simulink model "TestFilter"  (Simulink 6.6)
settings: Solver=ode45  StartTime=0.0  StopTime=10.0  RelTol=1e-3
undefined symbols (not defined in the file or in its folder): DiscIntNeverNeededParam, floatToBytes, gaind, polesd, u1, y1, zerosd
libraries: simulink x22, dsPICdrivers x15, aerolibguid x1, aerolibutil x1, dspmtrx3 x1
(part 1 of 2)
settings Model: Creator=ASL_Lab  LastModifiedBy=ASL_Lab

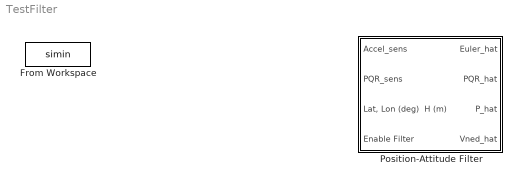
== system TestFilter ==
  From Workspace : FromWorkspace  VariableName=simin  SampleTime=0
  Position-Attitude Filter : Subsystem

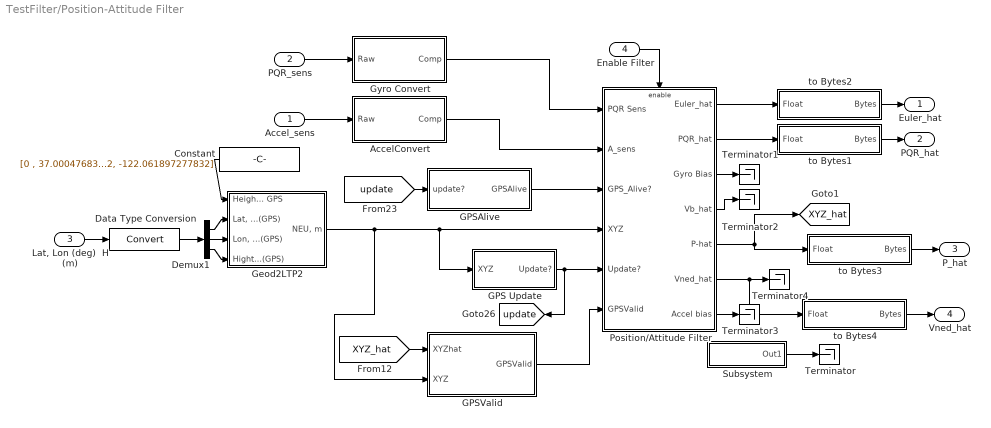
== system TestFilter/Position-Attitude Filter ==
  Accel_sens : Inport
  PQR_sens : Inport  Port=2
  "Lat, Lon (deg)  H (m)" : Inport  Port=3
  Enable Filter : Inport  Port=4
  AccelConvert : Subsystem  mask{bias=[2012 2018 2007], gains=[-41 41 -41]}
      mask prompts: bias "Initial Bias"; gains "Initial Gains"
      mask help: Convert Analog readings to units
  Constant : Constant  Orientation=left  Value=[0 , 37.0004768371582, -122.061897277832]
  Data Type Conversion : DataTypeConversion  OutDataTypeMode=double
  Demux1 : Demux  Outputs=3
  GPS Update : Subsystem  mask{T=0.01}
      mask prompts: T "Sample Time"
  GPSAlive : Subsystem  mask{deadLimit=4, T=0.01}
      mask prompts: deadLimit "Dead Limit (in Secs)"; T "Sample Time"
  GPSValid : Subsystem  mask{deadLimit=2000}
      mask prompts: deadLimit "Maximum Distance Error (in Mts)"
  Geod2LTP2 : Subsystem
      mask Description:
      | This block provides transformation of the Geodetic coordinates
      | to the LTP coorinate system. The block uses two consecutive transformations
      | (Geodetic -> ECEF ->LTP).
      | Geodetic coordinates of the LTP origin should also be predetermined.
      mask Help: Oops!
      mask Display: plot(0,0,100,100,[45,40,35,40,40],[85,95,85,95,40],[85,95,85,95,40],[35,40,45,40,40],[60,40,10,20,10,14],[70,40,10,13,10,20],[56,45],[70,70],[60,60],[50,60],[60,60],[30,40],[50,60],[20,20],[30,40],[20,20],[45,55],[35,25],[75,65],[35,25])
  Gyro Convert : Subsystem  mask{bias=[1863 2037 2040], gains=[-142 142 235]}
      mask prompts: bias "Initial Bias"; gains "Initial Gains"
      mask help: Convert Analog readings to units
  Position/Attitude Filter : Subsystem
  Subsystem : Subsystem
  Terminator{,1..4} (5 alike) : Terminator
  to Bytes1 : Subsystem
  to Bytes2 : Subsystem
  to Bytes3 : Subsystem
  to Bytes4 : Subsystem
  Euler_hat : Outport
  PQR_hat : Outport  Port=2
  P_hat : Outport  Port=3
  Vned_hat : Outport  Port=4
  tag scope: XYZ_hat=global, update=global
  wires:
  Enable Filter/1 -> Position/Attitude Filter/Enable
  Accel_sens/1 -> AccelConvert/1(Raw)
  PQR_sens/1 -> Gyro Convert/1(Raw)
  Geod2LTP2/1("NEU, m") -> GPS Update/1(XYZ), Position/Attitude Filter/4(XYZ), GPSValid/2(XYZ)
  "Lat, Lon (deg)  H (m)"/1 -> Data Type Conversion/1
  Demux1/3 -> Geod2LTP2/4(Hight,m(GPS))
  Demux1/2 -> Geod2LTP2/3("Lon, deg(GPS)")
  Demux1/1 -> Geod2LTP2/2("Lat, deg(GPS)")
  Constant/1 -> Geod2LTP2/1("Height, Lat, Lon Initials from GPS")
  GPSValid/1(GPSValid) -> Position/Attitude Filter/6(GPSValid)
  [XYZ_hat] -> GPSValid/1(XYZhat)
  GPSAlive/1(GPSAlive) -> Position/Attitude Filter/3(GPS_Alive?)
  [update] -> GPSAlive/1(update?)
  GPS Update/1(Update?) -> Position/Attitude Filter/5(Update?), [update]
  to Bytes2/1(Bytes) -> Euler_hat/1
  to Bytes1/1(Bytes) -> PQR_hat/1
  to Bytes3/1(Bytes) -> P_hat/1
  to Bytes4/1(Bytes) -> Vned_hat/1
  Subsystem/1(Out1) -> Terminator/1
  Position/Attitude Filter/5(P-hat) -> [XYZ_hat], to Bytes3/1(Float)
  Position/Attitude Filter/6(Vned_hat) -> Terminator4/1, to Bytes4/1(Float)
  Position/Attitude Filter/3(Gyro Bias) -> Terminator1/1
  Position/Attitude Filter/4(Vb_hat) -> Terminator2/1
  Position/Attitude Filter/7(Accel bias) -> Terminator3/1
  Position/Attitude Filter/1(Euler_hat) -> to Bytes2/1(Float)
  Position/Attitude Filter/2(PQR_hat) -> to Bytes1/1(Float)
  Gyro Convert/1(Comp) -> Position/Attitude Filter/1(PQR Sens)
  AccelConvert/1(Comp) -> Position/Attitude Filter/2(A_sens)
  Data Type Conversion/1 -> Demux1/1

== system TestFilter/Position-Attitude Filter/AccelConvert ==
  Raw : Inport
  Bias : Constant  Value=bias
  Divide : Product  Inputs=/*  OutScaling=2^-10
  Gains : Constant  Value=gains
  Sum : Sum  Inputs=|+-
  Comp : Outport
  wires:
  Raw/1 -> Sum/1
  Divide/1 -> Comp/1
  Sum/1 -> Divide/2
  Gains/1 -> Divide/1
  Bias/1 -> Sum/2

== system TestFilter/Position-Attitude Filter/GPS Update ==
  XYZ : Inport
  Demux : Demux  Outputs=3
  Detect Change : Subsystem
  Detect Change1 : Subsystem
  Detect Change2 : Subsystem
  Rate Transition : RateTransition  OutPortSampleTime=T
  Saturation1 : Saturate  UpperLimit=1  LowerLimit=0  SampleTime=T
  Sum : Sum  Inputs=3
  Update? : Outport
  wires:
  Rate Transition/1 -> Demux/1
  Saturation1/1 -> Update?/1
  XYZ/1 -> Rate Transition/1
  Sum/1 -> Saturation1/1
  Detect Change2/1(change?) -> Sum/3
  Detect Change1/1(change?) -> Sum/2
  Detect Change/1(change?) -> Sum/1
  Demux/3 -> Detect Change2/1(Data)
  Demux/2 -> Detect Change1/1(Data)
  Demux/1 -> Detect Change/1(Data)

== system TestFilter/Position-Attitude Filter/GPSAlive ==
  update? : Inport
  Compare To Constant : simulink/Logic and Bit Operations/Compare To Constant  SystemSampleTime=-1  relop=<=  const=deadLimit  LogicOutDataTypeMode=uint8  ZeroCross=off
  Constant : Constant
  Constant1 : Constant  Value=0
  Constant2 : Constant  Value=T
  Discrete-Time Integrator : DiscreteIntegrator  ExternalReset=rising  InitialConditionSource=external  SampleTime=T  ICPrevOutput=DiscIntNeverNeededParam  ICPrevScaledInput=DiscIntNeverNeededParam
  Integer Delay2 : simulink/Discrete/Integer Delay  vinit=0.0  samptime=-1  NumDelays=1
  Sum : Sum  Inputs=|++
  GPSAlive : Outport
  wires:
  Compare To Constant/1 -> GPSAlive/1
  Sum/1 -> Compare To Constant/1
  Constant2/1 -> Sum/2
  Integer Delay2/1 -> Sum/1
  update?/1 -> Discrete-Time Integrator/2
  Discrete-Time Integrator/1 -> Integer Delay2/1
  Constant1/1 -> Discrete-Time Integrator/3
  Constant/1 -> Discrete-Time Integrator/1

== system TestFilter/Position-Attitude Filter/GPSValid ==
  XYZhat : Inport
  XYZ : Inport  Port=2
  Calculate Range : aerolibguid/Calculate Range  SystemSampleTime=-1
  Compare To Constant : simulink/Logic and Bit Operations/Compare To Constant  SystemSampleTime=-1  relop=<=  const=deadLimit  LogicOutDataTypeMode=uint8  ZeroCross=off
  Integer Delay : simulink/Discrete/Integer Delay  vinit=0.0  samptime=0.01  NumDelays=1
  GPSValid : Outport
  wires:
  XYZ/1 -> Calculate Range/2
  Compare To Constant/1 -> GPSValid/1
  XYZhat/1 -> Integer Delay/1
  Calculate Range/1 -> Compare To Constant/1
  Integer Delay/1 -> Calculate Range/1

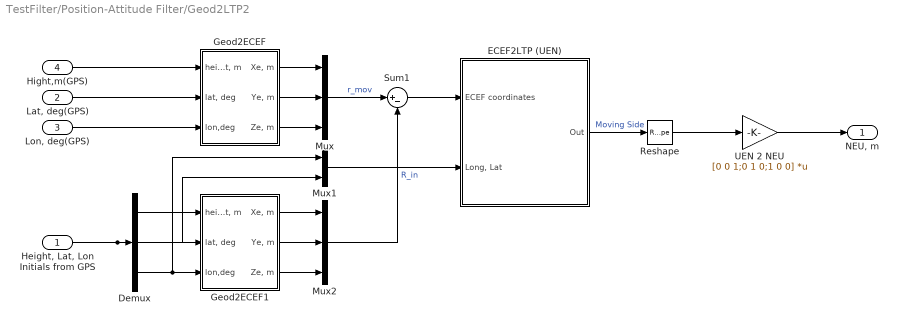
== system TestFilter/Position-Attitude Filter/Geod2LTP2 ==
  "Height, Lat, Lon Initials from GPS" : Inport
  "Lat, deg(GPS)" : Inport  Port=2
  "Lon, deg(GPS)" : Inport  Port=3
  Hight,m(GPS) : Inport  Port=4
  Demux : Demux  Outputs=3
  ECEF2LTP (UEN) : Subsystem
      mask Display: plot(0,0,100,100,[45,40,35,40,40],[85,95,85,95,40],[85,95,85,95,40],[35,40,45,40,40],[60,40,10,20,10,14],[70,40,10,13,10,20],[56,45],[70,70],[60,60],[50,60],[60,60],[30,40],[50,60],[20,20],[30,40],[20,20],[45,55],[35,25],[75,65],[35,25])
  Geod2ECEF : Subsystem  mask{Re=6378137, Rp=6356752.3142}
      mask prompts: Re "Enter equatorial radius, m"; Rp "Enter polar radius,m"
  Geod2ECEF1 : Subsystem  mask{Re=6378137, Rp=6356752.3142}
      mask prompts: Re "Enter equatorial radius, m"; Rp "Enter polar radius,m"
  Mux : Mux  Inputs=3
  Mux1 : Mux  Inputs=2
  Mux2 : Mux  Inputs=3
  Reshape : Reshape  OutputDimensionality=Column vector (2-D)
  Sum1 : Sum  Inputs=|+-  SaturateOnIntegerOverflow=on
  UEN 2 NEU : Gain  Gain=[0 0 1;0 1 0;1 0 0]  Multiplication=Matrix(K*u)  SaturateOnIntegerOverflow=on
  "NEU, m" : Outport
  wires:
  UEN 2 NEU/1 -> "NEU, m"/1
  Geod2ECEF/3("Ze, m ") -> Mux/3
  Geod2ECEF/1("Xe, m ") -> Mux/1
  Geod2ECEF/2("Ye, m ") -> Mux/2
  "Lat, deg(GPS)"/1 -> Geod2ECEF/2("lat, deg")
  "Lon, deg(GPS)"/1 -> Geod2ECEF/3(lon,deg)
  Mux1/1 -> ECEF2LTP (UEN)/2("Long, Lat")
  Geod2ECEF1/3("Ze, m ") -> Mux2/3
  Geod2ECEF1/1("Xe, m ") -> Mux2/1
  Geod2ECEF1/2("Ye, m ") -> Mux2/2
  Mux2/1 -> Sum1/2  "R_in"
  Demux/1 -> Geod2ECEF1/1("height, m")
  Demux/2 -> Mux1/2, Geod2ECEF1/2("lat, deg")
  Demux/3 -> Mux1/1, Geod2ECEF1/3(lon,deg)
  ECEF2LTP (UEN)/1(Out) -> Reshape/1  "Moving Side"
  Hight,m(GPS)/1 -> Geod2ECEF/1("height, m")
  "Height, Lat, Lon Initials from GPS"/1 -> Demux/1
  Mux/1 -> Sum1/1  "r_mov"
  Sum1/1 -> ECEF2LTP (UEN)/1(ECEF coordinates)
  Reshape/1 -> UEN 2 NEU/1

== system TestFilter/Position-Attitude Filter/Gyro Convert ==
  Raw : Inport
  Bias : Constant  Value=bias
  Divide : Product  Inputs=/*  OutScaling=2^-10
  Gains : Constant  Value=gains
  Sum : Sum  Inputs=|+-
  Comp : Outport
  wires:
  Bias/1 -> Sum/2
  Gains/1 -> Divide/1
  Sum/1 -> Divide/2
  Divide/1 -> Comp/1
  Raw/1 -> Sum/1

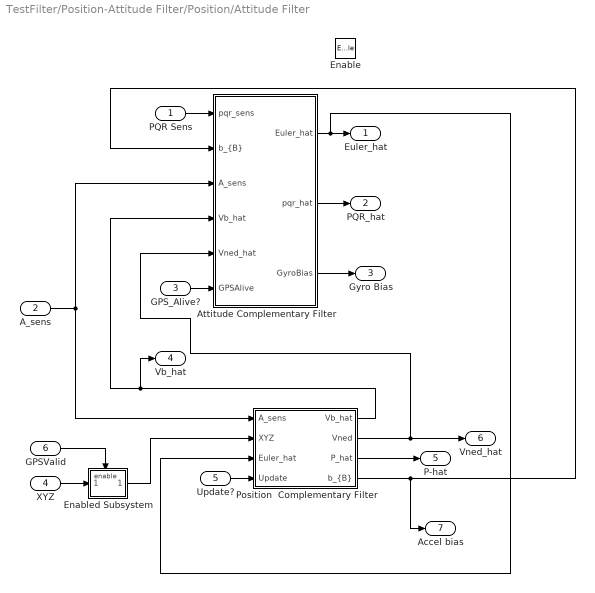
== system TestFilter/Position-Attitude Filter/Position/Attitude Filter ==
  PQR Sens : Inport
  A_sens : Inport  Port=2
  GPS_Alive? : Inport  Port=3
  XYZ : Inport  Port=4
  Update? : Inport  Port=5
  GPSValid : Inport  Port=6
  Enable : EnablePort  StatesWhenEnabling=reset
  Attitude Complementary Filter : Subsystem  mask{K1=0.7, K2=0.05, T=0.01, P0=[0 0 0], flpf=1}
      mask prompts: K1 "Euler Gain K1"; K2 "Bias Gain K2"; T "Filter Execution Time"; P0 "Initial Euler"; flpf "Feedback Low Pass Filter Freq (In S Domain)"
      mask help: Attitude Complementary filter based on the Magneto-Pendular Sensor by Vasconcelos, et.al.
      mask Help: Help
  Enabled Subsystem : Subsystem  TreatAsAtomicUnit=on
  Position  Complementary Filter : Subsystem  mask{K1=1.5, K2=0.5, K3=0.001, T=0.01, P0=[ 0 0 0], flpf=10}
      mask prompts: K1 "Position Gain K1"; K2 "Velocity Gain K2"; K3 "Bias Gain K3"; T "Filter Execution Time"; P0 "Initial Position"; flpf "Feedback Lowpass Filter Freq (in S domain)"
      mask help: Position Complementary filter based on the Magneto-Pendular Sensor by Vasconcelos, et.al.
      mask Help: Help
  Euler_hat : Outport
  PQR_hat : Outport  Port=2
  Gyro Bias : Outport  Port=3
  Vb_hat : Outport  Port=4
  P-hat : Outport  Port=5
  Vned_hat : Outport  Port=6
  Accel bias : Outport  Port=7
  wires:
  PQR Sens/1 -> Attitude Complementary Filter/1(pqr_sens)
  Attitude Complementary Filter/1(Euler_hat) -> Euler_hat/1, Position  Complementary Filter/3(Euler_hat)
  Attitude Complementary Filter/2(pqr_hat) -> PQR_hat/1
  A_sens/1 -> Attitude Complementary Filter/3(A_sens), Position  Complementary Filter/1(A_sens)
  Attitude Complementary Filter/3(GyroBias) -> Gyro Bias/1
  GPS_Alive?/1 -> Attitude Complementary Filter/6(GPSAlive)
  Position  Complementary Filter/1(Vb_hat) -> Attitude Complementary Filter/4(Vb_hat), Vb_hat/1
  Position  Complementary Filter/3(P_hat) -> P-hat/1
  Update?/1 -> Position  Complementary Filter/4(Update)
  Position  Complementary Filter/4("b_{B}") -> Accel bias/1, Attitude Complementary Filter/2("b_{B}")
  Position  Complementary Filter/2(Vned) -> Attitude Complementary Filter/5(Vned_hat), Vned_hat/1
  Enabled Subsystem/1(Out1) -> Position  Complementary Filter/2(XYZ)
  XYZ/1 -> Enabled Subsystem/1(In1)
  GPSValid/1 -> Enabled Subsystem/Enable

== system TestFilter/Position-Attitude Filter/Subsystem ==
  Mux : Mux  Inputs=3
  Sine Wave : Sin  SineType=Sample based  Amplitude=5*pi/180  Samples=100  SampleTime=.01
  Sine Wave1 : Sin  SineType=Sample based  Amplitude=10*pi/180  Samples=100  SampleTime=.01
  Sine Wave2 : Sin  SineType=Sample based  Amplitude=15*pi/180  Samples=100  SampleTime=.01
  Out1 : Outport
  wires:
  Sine Wave/1 -> Mux/1
  Sine Wave1/1 -> Mux/2
  Sine Wave2/1 -> Mux/3
  Mux/1 -> Out1/1

== system TestFilter/Position-Attitude Filter/to Bytes1 ==
  Float : Inport
  C Function Call : dsPICdrivers/OTHERS/C Function Call  Tag=dsPIC_dsPIC_CFunctionCall  fctName='floatToBytes'  INPUT_SIZE=1  INPUT1=real32  INPUT2=--  INPUT3=--  OUTPUT_SIZE=4  OUTPUT1=uint8  SampleTime=-1  InputType=[ 7 ]  OutputType=[ 2 ]  FctDeclaration=extern void floatToBytes(real32_T u1,uint8_T* y1);  FctCall=floatToBytes(%u1, *%y1);  OrderingInOutPopup=None
  C Function Call1 : dsPICdrivers/OTHERS/C Function Call  Tag=dsPIC_dsPIC_CFunctionCall  fctName='floatToBytes'  INPUT_SIZE=1  INPUT1=real32  INPUT2=--  INPUT3=--  OUTPUT_SIZE=4  OUTPUT1=uint8  SampleTime=-1  InputType=[ 7 ]  OutputType=[ 2 ]  FctDeclaration=extern void floatToBytes(real32_T u1,uint8_T* y1);  FctCall=floatToBytes(%u1, *%y1);  OrderingInOutPopup=None
  C Function Call2 : dsPICdrivers/OTHERS/C Function Call  Tag=dsPIC_dsPIC_CFunctionCall  fctName='floatToBytes'  INPUT_SIZE=1  INPUT1=real32  INPUT2=--  INPUT3=--  OUTPUT_SIZE=4  OUTPUT1=uint8  SampleTime=-1  InputType=[ 7 ]  OutputType=[ 2 ]  FctDeclaration=extern void floatToBytes(real32_T u1,uint8_T* y1);  FctCall=floatToBytes(%u1, *%y1);  OrderingInOutPopup=None
  Data Type Conversion : DataTypeConversion  OutDataTypeMode=single
  Demux : Demux  Outputs=3
  Mux : Mux  Inputs=3
  Bytes : Outport
  wires:
  Float/1 -> Data Type Conversion/1
  Demux/1 -> C Function Call/1
  Mux/1 -> Bytes/1
  C Function Call/1 -> Mux/1
  Demux/2 -> C Function Call1/1
  Demux/3 -> C Function Call2/1
  C Function Call1/1 -> Mux/2
  C Function Call2/1 -> Mux/3
  Data Type Conversion/1 -> Demux/1

== system TestFilter/Position-Attitude Filter/to Bytes2 ==
  Float : Inport
  C Function Call : dsPICdrivers/OTHERS/C Function Call  Tag=dsPIC_dsPIC_CFunctionCall  fctName='floatToBytes'  INPUT_SIZE=1  INPUT1=real32  INPUT2=--  INPUT3=--  OUTPUT_SIZE=4  OUTPUT1=uint8  SampleTime=-1  InputType=[ 7 ]  OutputType=[ 2 ]  FctDeclaration=extern void floatToBytes(real32_T u1,uint8_T* y1);  FctCall=floatToBytes(%u1, *%y1);  OrderingInOutPopup=None
  C Function Call1 : dsPICdrivers/OTHERS/C Function Call  Tag=dsPIC_dsPIC_CFunctionCall  fctName='floatToBytes'  INPUT_SIZE=1  INPUT1=real32  INPUT2=--  INPUT3=--  OUTPUT_SIZE=4  OUTPUT1=uint8  SampleTime=-1  InputType=[ 7 ]  OutputType=[ 2 ]  FctDeclaration=extern void floatToBytes(real32_T u1,uint8_T* y1);  FctCall=floatToBytes(%u1, *%y1);  OrderingInOutPopup=None
  C Function Call2 : dsPICdrivers/OTHERS/C Function Call  Tag=dsPIC_dsPIC_CFunctionCall  fctName='floatToBytes'  INPUT_SIZE=1  INPUT1=real32  INPUT2=--  INPUT3=--  OUTPUT_SIZE=4  OUTPUT1=uint8  SampleTime=-1  InputType=[ 7 ]  OutputType=[ 2 ]  FctDeclaration=extern void floatToBytes(real32_T u1,uint8_T* y1);  FctCall=floatToBytes(%u1, *%y1);  OrderingInOutPopup=None
  Data Type Conversion : DataTypeConversion  OutDataTypeMode=single
  Demux : Demux  Outputs=3
  Mux : Mux  Inputs=3
  Bytes : Outport
  wires:
  Data Type Conversion/1 -> Demux/1
  C Function Call2/1 -> Mux/3
  C Function Call1/1 -> Mux/2
  Demux/3 -> C Function Call2/1
  Demux/2 -> C Function Call1/1
  C Function Call/1 -> Mux/1
  Mux/1 -> Bytes/1
  Demux/1 -> C Function Call/1
  Float/1 -> Data Type Conversion/1

== system TestFilter/Position-Attitude Filter/to Bytes3 ==
  Float : Inport
  C Function Call : dsPICdrivers/OTHERS/C Function Call  Tag=dsPIC_dsPIC_CFunctionCall  fctName='floatToBytes'  INPUT_SIZE=1  INPUT1=real32  INPUT2=--  INPUT3=--  OUTPUT_SIZE=4  OUTPUT1=uint8  SampleTime=-1  InputType=[ 7 ]  OutputType=[ 2 ]  FctDeclaration=extern void floatToBytes(real32_T u1,uint8_T* y1);  FctCall=floatToBytes(%u1, *%y1);  OrderingInOutPopup=None
  C Function Call1 : dsPICdrivers/OTHERS/C Function Call  Tag=dsPIC_dsPIC_CFunctionCall  fctName='floatToBytes'  INPUT_SIZE=1  INPUT1=real32  INPUT2=--  INPUT3=--  OUTPUT_SIZE=4  OUTPUT1=uint8  SampleTime=-1  InputType=[ 7 ]  OutputType=[ 2 ]  FctDeclaration=extern void floatToBytes(real32_T u1,uint8_T* y1);  FctCall=floatToBytes(%u1, *%y1);  OrderingInOutPopup=None
  C Function Call2 : dsPICdrivers/OTHERS/C Function Call  Tag=dsPIC_dsPIC_CFunctionCall  fctName='floatToBytes'  INPUT_SIZE=1  INPUT1=real32  INPUT2=--  INPUT3=--  OUTPUT_SIZE=4  OUTPUT1=uint8  SampleTime=-1  InputType=[ 7 ]  OutputType=[ 2 ]  FctDeclaration=extern void floatToBytes(real32_T u1,uint8_T* y1);  FctCall=floatToBytes(%u1, *%y1);  OrderingInOutPopup=None
  Data Type Conversion : DataTypeConversion  OutDataTypeMode=single
  Demux : Demux  Outputs=3
  Mux : Mux  Inputs=3
  Bytes : Outport
  wires:
  Data Type Conversion/1 -> Demux/1
  C Function Call2/1 -> Mux/3
  C Function Call1/1 -> Mux/2
  Demux/3 -> C Function Call2/1
  Demux/2 -> C Function Call1/1
  C Function Call/1 -> Mux/1
  Mux/1 -> Bytes/1
  Demux/1 -> C Function Call/1
  Float/1 -> Data Type Conversion/1

== system TestFilter/Position-Attitude Filter/to Bytes4 ==
  Float : Inport
  C Function Call : dsPICdrivers/OTHERS/C Function Call  Tag=dsPIC_dsPIC_CFunctionCall  fctName='floatToBytes'  INPUT_SIZE=1  INPUT1=real32  INPUT2=--  INPUT3=--  OUTPUT_SIZE=4  OUTPUT1=uint8  SampleTime=-1  InputType=[ 7 ]  OutputType=[ 2 ]  FctDeclaration=extern void floatToBytes(real32_T u1,uint8_T* y1);  FctCall=floatToBytes(%u1, *%y1);  OrderingInOutPopup=None
  C Function Call1 : dsPICdrivers/OTHERS/C Function Call  Tag=dsPIC_dsPIC_CFunctionCall  fctName='floatToBytes'  INPUT_SIZE=1  INPUT1=real32  INPUT2=--  INPUT3=--  OUTPUT_SIZE=4  OUTPUT1=uint8  SampleTime=-1  InputType=[ 7 ]  OutputType=[ 2 ]  FctDeclaration=extern void floatToBytes(real32_T u1,uint8_T* y1);  FctCall=floatToBytes(%u1, *%y1);  OrderingInOutPopup=None
  C Function Call2 : dsPICdrivers/OTHERS/C Function Call  Tag=dsPIC_dsPIC_CFunctionCall  fctName='floatToBytes'  INPUT_SIZE=1  INPUT1=real32  INPUT2=--  INPUT3=--  OUTPUT_SIZE=4  OUTPUT1=uint8  SampleTime=-1  InputType=[ 7 ]  OutputType=[ 2 ]  FctDeclaration=extern void floatToBytes(real32_T u1,uint8_T* y1);  FctCall=floatToBytes(%u1, *%y1);  OrderingInOutPopup=None
  Data Type Conversion : DataTypeConversion  OutDataTypeMode=single
  Demux : Demux  Outputs=3
  Mux : Mux  Inputs=3
  Bytes : Outport
  wires:
  Float/1 -> Data Type Conversion/1
  Demux/1 -> C Function Call/1
  Mux/1 -> Bytes/1
  C Function Call/1 -> Mux/1
  Demux/2 -> C Function Call1/1
  Demux/3 -> C Function Call2/1
  C Function Call1/1 -> Mux/2
  C Function Call2/1 -> Mux/3
  Data Type Conversion/1 -> Demux/1

== system TestFilter/Position-Attitude Filter/GPS Update/Detect Change ==
  Data : Inport
  Abs1 : Abs  SampleTime=T
  Difference1 : simulink/Discrete/Difference  SystemSampleTime=-1  ICPrevInput=0.0  OutDataType=sfix(16)  OutScaling=2^-10  DoSatur=off
  Saturation1 : Saturate  UpperLimit=1  LowerLimit=0  SampleTime=T
  change? : Outport
  wires:
  Saturation1/1 -> change?/1
  Data/1 -> Difference1/1
  Abs1/1 -> Saturation1/1
  Difference1/1 -> Abs1/1

== system TestFilter/Position-Attitude Filter/GPS Update/Detect Change1 ==
  Data : Inport
  Abs1 : Abs  SampleTime=T
  Difference1 : simulink/Discrete/Difference  SystemSampleTime=-1  ICPrevInput=0.0  OutDataType=sfix(16)  OutScaling=2^-10  DoSatur=off
  Saturation1 : Saturate  UpperLimit=1  LowerLimit=0  SampleTime=T
  change? : Outport
  wires:
  Difference1/1 -> Abs1/1
  Abs1/1 -> Saturation1/1
  Data/1 -> Difference1/1
  Saturation1/1 -> change?/1

== system TestFilter/Position-Attitude Filter/GPS Update/Detect Change2 ==
  Data : Inport
  Abs1 : Abs  SampleTime=T
  Difference1 : simulink/Discrete/Difference  SystemSampleTime=-1  ICPrevInput=0.0  OutDataType=sfix(16)  OutScaling=2^-10  DoSatur=off
  Saturation1 : Saturate  UpperLimit=1  LowerLimit=0  SampleTime=T
  change? : Outport
  wires:
  Saturation1/1 -> change?/1
  Data/1 -> Difference1/1
  Abs1/1 -> Saturation1/1
  Difference1/1 -> Abs1/1

== system TestFilter/Position-Attitude Filter/Geod2LTP2/ECEF2LTP (UEN) ==
  ECEF coordinates : Inport
  "Long, Lat" : Inport  Port=2
  Deg2R : Gain  Gain=pi/180  SaturateOnIntegerOverflow=on
  Demux3 : Demux  Outputs=2
  From Body to Universal1 : Subsystem
  Product1 : Product  Multiplication=Matrix(*)  SaturateOnIntegerOverflow=on  InputSameDT=on
  Out : Outport
  wires:
  "Long, Lat"/1 -> Deg2R/1
  Product1/1 -> Out/1
  Demux3/2 -> From Body to Universal1/2(lat)
  Demux3/1 -> From Body to Universal1/1(long)
  Deg2R/1 -> Demux3/1
  ECEF coordinates/1 -> Product1/2
  From Body to Universal1/1(DCM) -> Product1/1

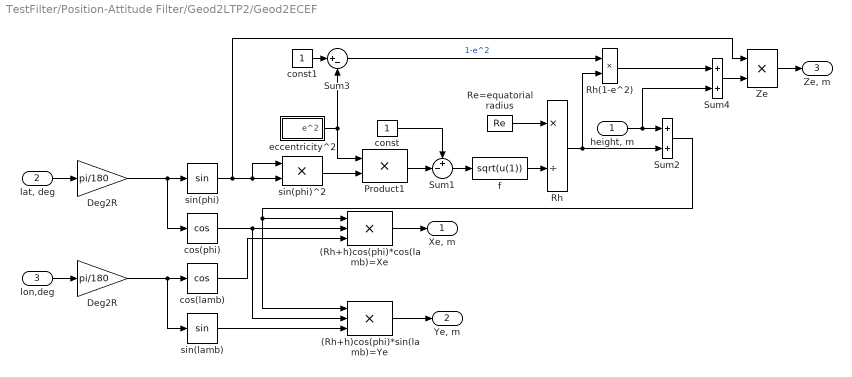
== system TestFilter/Position-Attitude Filter/Geod2LTP2/Geod2ECEF ==
  "height, m" : Inport
  "lat, deg" : Inport  Port=2
  lon,deg : Inport  Port=3
  (Rh+h)cos(phi)*cos(lamb)=Xe : Product  Inputs=3  SaturateOnIntegerOverflow=on  InputSameDT=on
  (Rh+h)cos(phi)*sin(lamb)=Ye : Product  Inputs=3  SaturateOnIntegerOverflow=on  InputSameDT=on
  Deg2R : Gain  Gain=pi/180  SaturateOnIntegerOverflow=on
  "Deg2R " : Gain  Gain=pi/180  SaturateOnIntegerOverflow=on
  Product1 : Product  SaturateOnIntegerOverflow=on  InputSameDT=on
  Re=equatorial radius : Constant  Value=Re
  Rh : Product  Inputs=*/  SaturateOnIntegerOverflow=on  InputSameDT=on
  Rh(1-e^2) : Product  SaturateOnIntegerOverflow=on  InputSameDT=on
  Sum1 : Sum  Inputs=+-|  SaturateOnIntegerOverflow=on  InputSameDT=on
  Sum2 : Sum  SaturateOnIntegerOverflow=on  InputSameDT=on
      settings: AttributesFormatString=Rh+h
  Sum3 : Sum  Inputs=|+-  SaturateOnIntegerOverflow=on  InputSameDT=on
  Sum4 : Sum  SaturateOnIntegerOverflow=on  InputSameDT=on
      settings: AttributesFormatString=(1-e^2)Rh+h
  Ze : Product  SaturateOnIntegerOverflow=on  InputSameDT=on
  const : Constant
  const1 : Constant
  cos(lamb) : Trigonometry  Operator=cos
  cos(phi) : Trigonometry  Operator=cos
  eccentricity^2 : Subsystem
  f : Fcn  Expr=sqrt(u(1))
  sin(lamb) : Trigonometry
  sin(phi) : Trigonometry
  sin(phi)^2 : Product  SaturateOnIntegerOverflow=on  InputSameDT=on
  "Xe, m " : Outport
  "Ye, m " : Outport  Port=2
  "Ze, m " : Outport  Port=3
  wires:
  "lat, deg"/1 -> Deg2R/1
  sin(phi)/1 -> sin(phi)^2/1, sin(phi)^2/2, Ze/1
  f/1 -> Rh/2
  Re=equatorial radius/1 -> Rh/1
  Rh/1 -> Sum2/2, Rh(1-e^2)/2
  Product1/1 -> Sum1/2
  Sum1/1 -> f/1
  const/1 -> Sum1/1
  "height, m"/1 -> Sum4/2, Sum2/1
  eccentricity^2/1(e^2) -> Product1/1, Sum3/2
  sin(phi)^2/1 -> Product1/2
  const1/1 -> Sum3/1
  Sum3/1 -> Rh(1-e^2)/1  "1-e^2"
  Rh(1-e^2)/1 -> Sum4/1
  Sum4/1 -> Ze/2
  lon,deg/1 -> "Deg2R "/1
  cos(phi)/1 -> (Rh+h)cos(phi)*cos(lamb)=Xe/2, (Rh+h)cos(phi)*sin(lamb)=Ye/2
  cos(lamb)/1 -> (Rh+h)cos(phi)*cos(lamb)=Xe/3
  sin(lamb)/1 -> (Rh+h)cos(phi)*sin(lamb)=Ye/3
  Ze/1 -> "Ze, m "/1
  Deg2R/1 -> cos(phi)/1, sin(phi)/1
  "Deg2R "/1 -> cos(lamb)/1, sin(lamb)/1
  Sum2/1 -> (Rh+h)cos(phi)*sin(lamb)=Ye/1, (Rh+h)cos(phi)*cos(lamb)=Xe/1
  (Rh+h)cos(phi)*cos(lamb)=Xe/1 -> "Xe, m "/1
  (Rh+h)cos(phi)*sin(lamb)=Ye/1 -> "Ye, m "/1

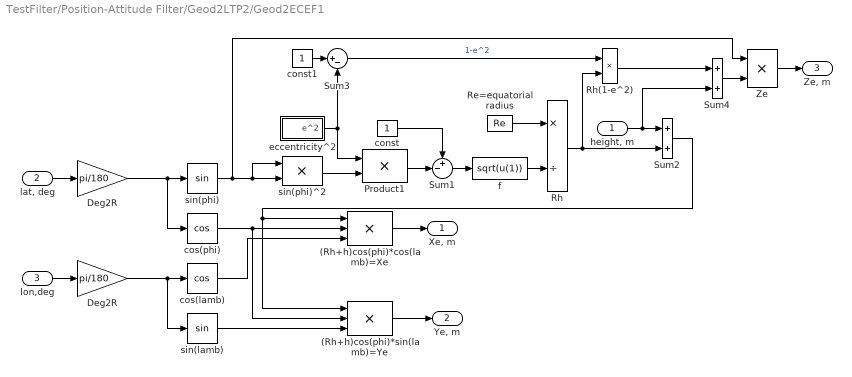
== system TestFilter/Position-Attitude Filter/Geod2LTP2/Geod2ECEF1 ==
  "height, m" : Inport
  "lat, deg" : Inport  Port=2
  lon,deg : Inport  Port=3
  (Rh+h)cos(phi)*cos(lamb)=Xe : Product  Inputs=3  SaturateOnIntegerOverflow=on  InputSameDT=on
  (Rh+h)cos(phi)*sin(lamb)=Ye : Product  Inputs=3  SaturateOnIntegerOverflow=on  InputSameDT=on
  Deg2R : Gain  Gain=pi/180  SaturateOnIntegerOverflow=on
  "Deg2R " : Gain  Gain=pi/180  SaturateOnIntegerOverflow=on
  Product1 : Product  SaturateOnIntegerOverflow=on  InputSameDT=on
  Re=equatorial radius : Constant  Value=Re
  Rh : Product  Inputs=*/  SaturateOnIntegerOverflow=on  InputSameDT=on
  Rh(1-e^2) : Product  SaturateOnIntegerOverflow=on  InputSameDT=on
  Sum1 : Sum  Inputs=+-|  SaturateOnIntegerOverflow=on  InputSameDT=on
  Sum2 : Sum  SaturateOnIntegerOverflow=on  InputSameDT=on
      settings: AttributesFormatString=Rh+h
  Sum3 : Sum  Inputs=|+-  SaturateOnIntegerOverflow=on  InputSameDT=on
  Sum4 : Sum  SaturateOnIntegerOverflow=on  InputSameDT=on
      settings: AttributesFormatString=(1-e^2)Rh+h
  Ze : Product  SaturateOnIntegerOverflow=on  InputSameDT=on
  const : Constant
  const1 : Constant
  cos(lamb) : Trigonometry  Operator=cos
  cos(phi) : Trigonometry  Operator=cos
  eccentricity^2 : Subsystem
  f : Fcn  Expr=sqrt(u(1))
  sin(lamb) : Trigonometry
  sin(phi) : Trigonometry
  sin(phi)^2 : Product  SaturateOnIntegerOverflow=on  InputSameDT=on
  "Xe, m " : Outport
  "Ye, m " : Outport  Port=2
  "Ze, m " : Outport  Port=3
  wires:
  (Rh+h)cos(phi)*sin(lamb)=Ye/1 -> "Ye, m "/1
  (Rh+h)cos(phi)*cos(lamb)=Xe/1 -> "Xe, m "/1
  Sum2/1 -> (Rh+h)cos(phi)*cos(lamb)=Xe/1, (Rh+h)cos(phi)*sin(lamb)=Ye/1
  "Deg2R "/1 -> sin(lamb)/1, cos(lamb)/1
  Deg2R/1 -> sin(phi)/1, cos(phi)/1
  Ze/1 -> "Ze, m "/1
  sin(lamb)/1 -> (Rh+h)cos(phi)*sin(lamb)=Ye/3
  cos(lamb)/1 -> (Rh+h)cos(phi)*cos(lamb)=Xe/3
  cos(phi)/1 -> (Rh+h)cos(phi)*sin(lamb)=Ye/2, (Rh+h)cos(phi)*cos(lamb)=Xe/2
  lon,deg/1 -> "Deg2R "/1
  Sum4/1 -> Ze/2
  Rh(1-e^2)/1 -> Sum4/1
  Sum3/1 -> Rh(1-e^2)/1  "1-e^2"
  const1/1 -> Sum3/1
  sin(phi)^2/1 -> Product1/2
  eccentricity^2/1(e^2) -> Sum3/2, Product1/1
  "height, m"/1 -> Sum2/1, Sum4/2
  const/1 -> Sum1/1
  Sum1/1 -> f/1
  Product1/1 -> Sum1/2
  Rh/1 -> Rh(1-e^2)/2, Sum2/2
  Re=equatorial radius/1 -> Rh/1
  f/1 -> Rh/2
  sin(phi)/1 -> Ze/1, sin(phi)^2/2, sin(phi)^2/1
  "lat, deg"/1 -> Deg2R/1

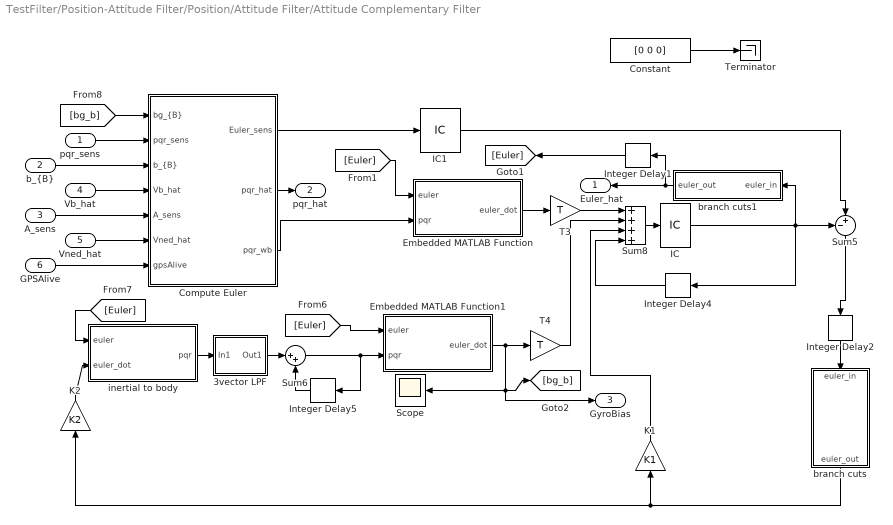
== system TestFilter/Position-Attitude Filter/Position/Attitude Filter/Attitude Complementary Filter ==
  pqr_sens : Inport
  "b_{B}" : Inport  Port=2
  A_sens : Inport  Port=3
  Vb_hat : Inport  Port=4
  Vned_hat : Inport  Port=5
  GPSAlive : Inport  Port=6
  3vector LPF : Subsystem  mask{flpf=flpf, T=T}
      mask prompts: flpf "Low Pass Frequency (in S domain)"; T "Sample time"
      mask Display: droots([],-flpf,flpf)
  Compute Euler : Subsystem
  Constant : Constant  Value=[0 0 0]
  Embedded MATLAB Function : Stateflow chart
  Embedded MATLAB Function1 : Stateflow chart
  IC : InitialCondition  Value=P0  SampleTime=T
  IC1 : InitialCondition  Value=P0  SampleTime=T
  Integer Delay1 : simulink/Discrete/Integer Delay  Orientation=left  vinit=0.0  samptime=-1  NumDelays=1
  Integer Delay2 : simulink/Discrete/Integer Delay  Orientation=down  vinit=0.0  samptime=-1  NumDelays=1
  Integer Delay4 : simulink/Discrete/Integer Delay  Orientation=left  vinit=0.0  samptime=-1  NumDelays=1
  Integer Delay5 : simulink/Discrete/Integer Delay  Orientation=left  vinit=0.0  samptime=-1  NumDelays=1
  K1 : Gain  Orientation=up  Gain=K1
  K2 : Gain  Orientation=up  Gain=K2
  Scope : Scope
      settings: TimeRange=60  YMin=-0.07116438310879042  YMax=0.01417979172834782  SaveName=ScopeData13
  Sum5 : Sum  Orientation=down  Inputs=-+|
  Sum6 : Sum  Inputs=|++
  Sum8 : Sum  Inputs=4
  T3 : Gain  Gain=T  SampleTime=T
  T4 : Gain  Gain=T  SampleTime=T
  Terminator : Terminator
  branch cuts : Stateflow chart  Orientation=down
  branch cuts1 : Stateflow chart  Orientation=left
  inertial to body : Stateflow chart
  Euler_hat : Outport  Orientation=left
  pqr_hat : Outport  Port=2
  GyroBias : Outport  Port=3
  wires:
  Embedded MATLAB Function/1(euler_dot) -> T3/1
  T3/1 -> Sum8/1
  Sum8/1 -> IC/1
  Integer Delay4/1 -> Sum8/4
  K1/1 -> Sum8/3
  inertial to body/1(pqr) -> 3vector LPF/1(In1)
  Sum6/1 -> Embedded MATLAB Function1/2(pqr), Integer Delay5/1
  [Euler] -> Embedded MATLAB Function1/1(euler)
  [Euler] -> inertial to body/1(euler)
  Embedded MATLAB Function1/1(euler_dot) -> [bg_b], Scope/1, GyroBias/1, T4/1
  T4/1 -> Sum8/2
  Integer Delay5/1 -> Sum6/2
  K2/1 -> inertial to body/2(euler_dot)
  [bg_b] -> Compute Euler/1("bg_{B}")
  pqr_sens/1 -> Compute Euler/2(pqr_sens)
  "b_{B}"/1 -> Compute Euler/3("b_{B}")
  Vb_hat/1 -> Compute Euler/4(Vb_hat)
  A_sens/1 -> Compute Euler/5(A_sens)
  Vned_hat/1 -> Compute Euler/6(Vned_hat)
  Sum5/1 -> Integer Delay2/1
  IC/1 -> Integer Delay4/1, Sum5/1, branch cuts1/1(euler_in)
  Integer Delay1/1 -> [Euler]
  [Euler] -> Embedded MATLAB Function/1(euler)
  Integer Delay2/1 -> branch cuts/1(euler_in)
  Compute Euler/3(pqr_wb) -> Embedded MATLAB Function/2(pqr)
  Compute Euler/2(pqr_hat) -> pqr_hat/1
  branch cuts/1(euler_out) -> K2/1, K1/1
  branch cuts1/1(euler_out) -> Euler_hat/1, Integer Delay1/1
  GPSAlive/1 -> Compute Euler/7(gpsAlive)
  3vector LPF/1(Out1) -> Sum6/1
  Compute Euler/1(Euler_sens) -> IC1/1
  IC1/1 -> Sum5/2
  Constant/1 -> Terminator/1

== system TestFilter/Position-Attitude Filter/Position/Attitude Filter/Enabled Subsystem ==
  In1 : Inport
  Enable : EnablePort
  Out1 : Outport
  wires:
  In1/1 -> Out1/1

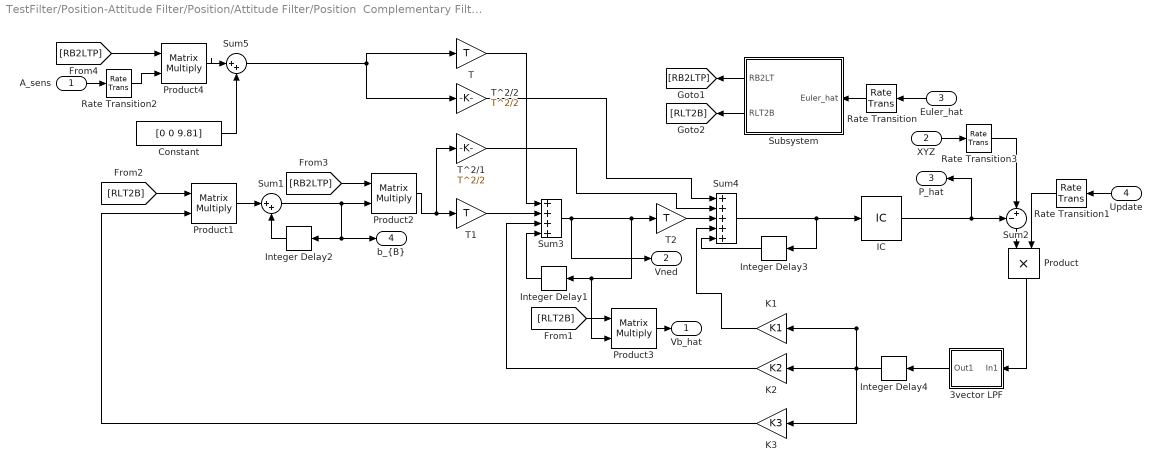
== system TestFilter/Position-Attitude Filter/Position/Attitude Filter/Position  Complementary Filter ==
  A_sens : Inport
  XYZ : Inport  Port=2
  Euler_hat : Inport  Orientation=left  Port=3
  Update : Inport  Orientation=left  Port=4
  3vector LPF : Subsystem  Orientation=left  mask{flpf=flpf, T=T}
      mask prompts: flpf "Low Pass Frequency (in S domain)"; T "Sample time"
      mask Display: droots([],-flpf,flpf)
  Constant : Constant  Value=[0 0 9.81]  SampleTime=0.01
  IC : InitialCondition  Value=P0  SampleTime=T
  Integer Delay{1..4} (4 alike) : simulink/Discrete/Integer Delay  Orientation=left  vinit=0.0  samptime=-1  NumDelays=1
  K1 : Gain  Orientation=left  Gain=K1
  K2 : Gain  Orientation=left  Gain=K2
  K3 : Gain  Orientation=left  Gain=K3
  Product : Product  Orientation=down  RndMeth=Zero
  Product{1..4} (4 alike) : Product  Multiplication=Matrix(*)  RndMeth=Zero
  Rate Transition : RateTransition  Orientation=left  OutPortSampleTime=T
  Rate Transition1 : RateTransition  Orientation=left  OutPortSampleTime=T
  Rate Transition2 : RateTransition  OutPortSampleTime=T
  Rate Transition3 : RateTransition  OutPortSampleTime=T
  Subsystem : Subsystem  Orientation=left
  Sum1 : Sum  Inputs=|++
  Sum2 : Sum  Orientation=down  Inputs=-+|
  Sum3 : Sum  Inputs=4
  Sum4 : Sum  Inputs=5
  Sum5 : Sum  Inputs=|++
  T : Gain  Gain=T
  T1 : Gain  Gain=T
  T2 : Gain  Gain=T
  T^2/1 : Gain  Gain=T^2/2
  T^2/2 : Gain  Gain=T^2/2
  Vb_hat : Outport
  Vned : Outport  Port=2
  P_hat : Outport  Orientation=left  Port=3
  "b_{B}" : Outport  Port=4
  wires:
  Subsystem/2(RLT2B) -> [RLT2B]
  Subsystem/1(RB2LT) -> [RB2LTP]
  Euler_hat/1 -> Rate Transition/1
  K3/1 -> Product1/2
  Product1/1 -> Sum1/1
  Sum1/1 -> Product2/2, Integer Delay2/1, "b_{B}"/1
  Product2/1 -> T^2/1/1, T1/1
  T1/1 -> Sum3/2
  T/1 -> Sum3/1
  Sum3/1 -> T2/1, Integer Delay1/1, Product3/2, Vned/1
  K2/1 -> Sum3/3
  T2/1 -> Sum4/3
  T^2/1/1 -> Sum4/2
  T^2/2/1 -> Sum4/1
  Sum4/1 -> Integer Delay3/1, IC/1
  K1/1 -> Sum4/4
  XYZ/1 -> Rate Transition3/1
  Product3/1 -> Vb_hat/1
  Sum2/1 -> Product/1
  Product/1 -> 3vector LPF/1(In1)
  Update/1 -> Rate Transition1/1
  Integer Delay3/1 -> Sum4/5
  Integer Delay2/1 -> Sum1/2
  Integer Delay1/1 -> Sum3/4
  A_sens/1 -> Rate Transition2/1
  Product4/1 -> Sum5/1
  Constant/1 -> Sum5/2
  Sum5/1 -> T/1, T^2/2/1
  Rate Transition/1 -> Subsystem/1(Euler_hat)
  Rate Transition1/1 -> Product/2
  Rate Transition3/1 -> Sum2/2
  [RLT2B] -> Product1/1
  [RB2LTP] -> Product4/1
  Rate Transition2/1 -> Product4/2
  [RB2LTP] -> Product2/1
  [RLT2B] -> Product3/1
  IC/1 -> Sum2/1, P_hat/1
  Integer Delay4/1 -> K1/1, K2/1, K3/1
  3vector LPF/1(Out1) -> Integer Delay4/1

== system TestFilter/Position-Attitude Filter/Geod2LTP2/ECEF2LTP (UEN)/From Body to Universal1 ==
  long : Inport
  lat : Inport  Port=2
  Mux : Mux  Inputs=2
  Reshape 9x1->3x1 : S-Function  FunctionName=sreshape  Parameters=OutputDimensionality, OutputDimensions  mask(Reshape){OutputDimensionality=Customize, OutputDimensions=[3,3]}
      mask prompts: OutputDimensionality "Output dimensionality:"; OutputDimensions "Output dimensions:"
      mask help:
      | Change the dimensions of a vector or matrix input signal. Output
      |  - a one-dimensional array (vector),
      |  - a column vector (Mx1 matrix),
      |  - a row vector (1xN matrix), or
      |  - a matrix or vector with specified dimensions, e.g., [M, N] or [W].
      mask init:
      | s = reshapemask(gcb,'init');
      mask StyleString: popup(1-D array|Column vector|Row vector|Customize),edit
      mask CallbackString: reshapemask(gcb,'cbDimensionality')|
      mask Display: disp('Reshape')
  Rotation Matrix from Long//Lat : Subsystem
      mask Type: Vector Transformation
      mask Description: Vector Transformation
      mask Display: disp('axis')
  DCM : Outport
  wires:
  lat/1 -> Mux/2
  long/1 -> Mux/1
  Mux/1 -> Rotation Matrix from Long//Lat/1(long lat)
  Rotation Matrix from Long//Lat/1(DCM) -> Reshape 9x1->3x1/1
  Reshape 9x1->3x1/1 -> DCM/1

== system TestFilter/Position-Attitude Filter/Geod2LTP2/Geod2ECEF/eccentricity^2 ==
  " " : Product  SaturateOnIntegerOverflow=on  InputSameDT=on
  Re=equatorial radius1 : Constant  Value=Re
  Rp=polar radius : Constant  Value=Rp
  Sum5 : Sum  Inputs=|+-  SaturateOnIntegerOverflow=on  InputSameDT=on
  const2 : Constant
  e^1 : Product  Inputs=*/  SaturateOnIntegerOverflow=on  InputSameDT=on
  e^2 : Outport
  wires:
  Re=equatorial radius1/1 -> e^1/2
  Rp=polar radius/1 -> e^1/1
  const2/1 -> Sum5/1
  e^1/1 -> " "/2, " "/1
  " "/1 -> Sum5/2
  Sum5/1 -> e^2/1

== system TestFilter/Position-Attitude Filter/Geod2LTP2/Geod2ECEF1/eccentricity^2 ==
  " " : Product  SaturateOnIntegerOverflow=on  InputSameDT=on
  Re=equatorial radius1 : Constant  Value=Re
  Rp=polar radius : Constant  Value=Rp
  Sum5 : Sum  Inputs=|+-  SaturateOnIntegerOverflow=on  InputSameDT=on
  const2 : Constant
  e^1 : Product  Inputs=*/  SaturateOnIntegerOverflow=on  InputSameDT=on
  e^2 : Outport
  wires:
  Sum5/1 -> e^2/1
  " "/1 -> Sum5/2
  e^1/1 -> " "/1, " "/2
  const2/1 -> Sum5/1
  Rp=polar radius/1 -> e^1/1
  Re=equatorial radius1/1 -> e^1/2

== system TestFilter/Position-Attitude Filter/Position/Attitude Filter/Attitude Complementary Filter/3vector LPF ==
  In1 : Inport  Orientation=left
  Demux : Demux  Orientation=left  Outputs=3
  Low Pass1 : Subsystem  Orientation=left  mask(DiscretizedZeroPole){Zeros=[], Poles=[-flpf], Gain=flpf, AbsTol=auto, SampleTime=T, method=tustin, Wc=1}
      mask prompts: Zeros "Zeros (enter in s-main:)"; Poles "Poles (enter in s-domain:)"; Gain "Gain (enter in s-domain:)"; AbsTol "Absolute tolerance:"; SampleTime "Sample time:"; Wc "Critical Frequency (Hz):"
      mask help: Continuous mask uses c2d to transform parameters onto the Discrete Zero-Pole block inside.
      mask init:
      | st=SampleTime;
      | if length(st)>1
      |     st=SampleTime(1);
      | end
      | if(st>0)
      |     [zerosd,polesd,gaind] = sldiscutil('disczpk', {st,method,Wc,Zeros,Poles,Gain});
      | end	
      | s = get_param(gcb,'maskvalues');
      | zeross = s{1};
      | poless = s{2};
      | gainss = s{3};
      | %zerosc = eval(zeross);
      | %polesc = eval(poless);
      | %gainsc = eval(gainss);
      | sldiscutil('initzpkmask', st);
      | if(st==0)
      | set_param([gcb '/Zero Pole'], 'AbsoluteTolerance', AbsTol);
      | end
      mask StyleString: edit,edit,edit,edit,edit,popup(zoh|foh|tustin|prewarp|matched),edit
      mask CallbackString: |||||hidecrit|
      mask Display:
      | droots(zeross,poless,gainss)
      | text( 0.5, 1.0, method, 'verticalAlignment','top')
  Low Pass2 : Subsystem  Orientation=left  mask(DiscretizedZeroPole){Zeros=[], Poles=[-flpf], Gain=flpf, AbsTol=auto, SampleTime=T, method=tustin, Wc=1}
      mask prompts: Zeros "Zeros (enter in s-main:)"; Poles "Poles (enter in s-domain:)"; Gain "Gain (enter in s-domain:)"; AbsTol "Absolute tolerance:"; SampleTime "Sample time:"; Wc "Critical Frequency (Hz):"
      mask help: Continuous mask uses c2d to transform parameters onto the Discrete Zero-Pole block inside.
      mask init: same as TestFilter/Position-Attitude Filter/Position/Attitude Filter/Attitude Complementary Filter/3vector LPF/Low Pass1
      mask StyleString: edit,edit,edit,edit,edit,popup(zoh|foh|tustin|prewarp|matched),edit
      mask CallbackString: |||||hidecrit|
      mask Display:
      | droots(zeross,poless,gainss)
      | text( 0.5, 1.0, method, 'verticalAlignment','top')
  Low Pass3 : Subsystem  Orientation=left  mask(DiscretizedZeroPole){Zeros=[], Poles=[-flpf], Gain=flpf, AbsTol=auto, SampleTime=T, method=tustin, Wc=1}
      mask prompts: Zeros "Zeros (enter in s-main:)"; Poles "Poles (enter in s-domain:)"; Gain "Gain (enter in s-domain:)"; AbsTol "Absolute tolerance:"; SampleTime "Sample time:"; Wc "Critical Frequency (Hz):"
      mask help: Continuous mask uses c2d to transform parameters onto the Discrete Zero-Pole block inside.
      mask init: same as TestFilter/Position-Attitude Filter/Position/Attitude Filter/Attitude Complementary Filter/3vector LPF/Low Pass1
      mask StyleString: edit,edit,edit,edit,edit,popup(zoh|foh|tustin|prewarp|matched),edit
      mask CallbackString: |||||hidecrit|
      mask Display:
      | droots(zeross,poless,gainss)
      | text( 0.5, 1.0, method, 'verticalAlignment','top')
  Mux : Mux  Orientation=left  Inputs=3
  Out1 : Outport  Orientation=left
  wires:
  Demux/1 -> Low Pass1/1(In1)
  Demux/2 -> Low Pass2/1(In1)
  Demux/3 -> Low Pass3/1(In1)
  Low Pass1/1(Out1) -> Mux/1
  Low Pass2/1(Out1) -> Mux/2
  Low Pass3/1(Out1) -> Mux/3
  In1/1 -> Demux/1
  Mux/1 -> Out1/1

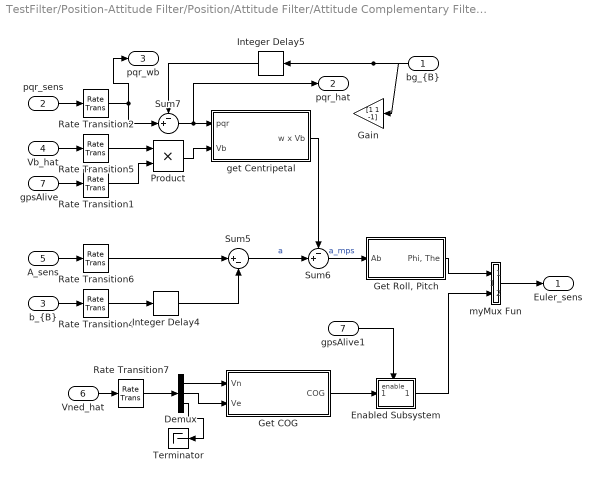
== system TestFilter/Position-Attitude Filter/Position/Attitude Filter/Attitude Complementary Filter/Compute Euler ==
  "bg_{B}" : Inport  Orientation=left
  pqr_sens : Inport  Port=2
  "b_{B}" : Inport  Port=3
  Vb_hat : Inport  Port=4
  A_sens : Inport  Port=5
  Vned_hat : Inport  Port=6
  gpsAlive : Inport  Port=7
  Demux : Demux  Outputs=3
  Enabled Subsystem : Subsystem  TreatAsAtomicUnit=on
  Gain : Gain  Orientation=left  Gain=[1 1 -1]
  Get COG : Subsystem
  "Get Roll, Pitch" : Subsystem
  Integer Delay4 : simulink/Discrete/Integer Delay  vinit=0.0  samptime=-1  NumDelays=1
  Integer Delay5 : simulink/Discrete/Integer Delay  Orientation=left  vinit=0.0  samptime=-1  NumDelays=1
  Product : Product  RndMeth=Zero
  Rate Transition{1..2,4..7} (6 alike) : RateTransition  OutPortSampleTime=T
  Sum5 : Sum  Inputs=|+-
  Sum6 : Sum  Inputs=-+|
  Sum7 : Sum  Inputs=-+|
  Terminator : Terminator
  get Centripetal : Subsystem
  gpsAlive1 : InportShadow  Port=7  LatchByCopyingInsideSignal=off
  myMux Fun : Stateflow chart
  Euler_sens : Outport
  pqr_hat : Outport  Port=2
  pqr_wb : Outport  Port=3
  wires:
  pqr_sens/1 -> Rate Transition2/1
  "b_{B}"/1 -> Rate Transition4/1
  Integer Delay4/1 -> Sum5/2
  Rate Transition6/1 -> Sum5/1
  Rate Transition4/1 -> Integer Delay4/1
  Vb_hat/1 -> Rate Transition5/1
  A_sens/1 -> Rate Transition6/1
  Sum5/1 -> Sum6/2  "a"
  Sum6/1 -> "Get Roll, Pitch"/1(Ab)  "a_mps"
  Rate Transition2/1 -> Sum7/2, pqr_wb/1
  Sum7/1 -> get Centripetal/1(pqr), pqr_hat/1
  Vned_hat/1 -> Rate Transition7/1
  "Get Roll, Pitch"/1("Phi, The") -> myMux Fun/1(u1)
  "bg_{B}"/1 -> Integer Delay5/1, Gain/1
  myMux Fun/1(y) -> Euler_sens/1
  get Centripetal/1(w x Vb) -> Sum6/1
  Rate Transition7/1 -> Demux/1
  Demux/1 -> Get COG/1(Vn)
  Demux/2 -> Get COG/2(Ve)
  Demux/3 -> Terminator/1
  Integer Delay5/1 -> Sum7/1
  gpsAlive/1 -> Rate Transition1/1
  Rate Transition1/1 -> Product/2
  Rate Transition5/1 -> Product/1
  Product/1 -> get Centripetal/2(Vb)
  Get COG/1(COG) -> Enabled Subsystem/1(In1)
  Enabled Subsystem/1(Out1) -> myMux Fun/2(u2)
  gpsAlive1/1 -> Enabled Subsystem/Enable

== system TestFilter/Position-Attitude Filter/Position/Attitude Filter/Position  Complementary Filter/3vector LPF ==
  In1 : Inport  Orientation=left
  Demux : Demux  Orientation=left  Outputs=3
  Low Pass1 : Subsystem  Orientation=left  mask(DiscretizedZeroPole){Zeros=[], Poles=[-flpf], Gain=flpf, AbsTol=auto, SampleTime=T, method=tustin, Wc=1}
      mask prompts: Zeros "Zeros (enter in s-main:)"; Poles "Poles (enter in s-domain:)"; Gain "Gain (enter in s-domain:)"; AbsTol "Absolute tolerance:"; SampleTime "Sample time:"; Wc "Critical Frequency (Hz):"
      mask help: Continuous mask uses c2d to transform parameters onto the Discrete Zero-Pole block inside.
      mask init: same as TestFilter/Position-Attitude Filter/Position/Attitude Filter/Attitude Complementary Filter/3vector LPF/Low Pass1
      mask StyleString: edit,edit,edit,edit,edit,popup(zoh|foh|tustin|prewarp|matched),edit
      mask CallbackString: |||||hidecrit|
      mask Display:
      | droots(zeross,poless,gainss)
      | text( 0.5, 1.0, method, 'verticalAlignment','top')
  Low Pass2 : Subsystem  Orientation=left  mask(DiscretizedZeroPole){Zeros=[], Poles=[-flpf], Gain=flpf, AbsTol=auto, SampleTime=T, method=tustin, Wc=1}
      mask prompts: Zeros "Zeros (enter in s-main:)"; Poles "Poles (enter in s-domain:)"; Gain "Gain (enter in s-domain:)"; AbsTol "Absolute tolerance:"; SampleTime "Sample time:"; Wc "Critical Frequency (Hz):"
      mask help: Continuous mask uses c2d to transform parameters onto the Discrete Zero-Pole block inside.
      mask init: same as TestFilter/Position-Attitude Filter/Position/Attitude Filter/Attitude Complementary Filter/3vector LPF/Low Pass1
      mask StyleString: edit,edit,edit,edit,edit,popup(zoh|foh|tustin|prewarp|matched),edit
      mask CallbackString: |||||hidecrit|
      mask Display:
      | droots(zeross,poless,gainss)
      | text( 0.5, 1.0, method, 'verticalAlignment','top')
  Low Pass3 : Subsystem  Orientation=left  mask(DiscretizedZeroPole){Zeros=[], Poles=[-flpf], Gain=flpf, AbsTol=auto, SampleTime=T, method=tustin, Wc=1}
      mask prompts: Zeros "Zeros (enter in s-main:)"; Poles "Poles (enter in s-domain:)"; Gain "Gain (enter in s-domain:)"; AbsTol "Absolute tolerance:"; SampleTime "Sample time:"; Wc "Critical Frequency (Hz):"
      mask help: Continuous mask uses c2d to transform parameters onto the Discrete Zero-Pole block inside.
      mask init: same as TestFilter/Position-Attitude Filter/Position/Attitude Filter/Attitude Complementary Filter/3vector LPF/Low Pass1
      mask StyleString: edit,edit,edit,edit,edit,popup(zoh|foh|tustin|prewarp|matched),edit
      mask CallbackString: |||||hidecrit|
      mask Display:
      | droots(zeross,poless,gainss)
      | text( 0.5, 1.0, method, 'verticalAlignment','top')
  Mux : Mux  Orientation=left  Inputs=3
  Out1 : Outport  Orientation=left
  wires:
  Demux/1 -> Low Pass1/1(In1)
  Demux/2 -> Low Pass2/1(In1)
  Demux/3 -> Low Pass3/1(In1)
  Low Pass1/1(Out1) -> Mux/1
  Low Pass2/1(Out1) -> Mux/2
  Low Pass3/1(Out1) -> Mux/3
  In1/1 -> Demux/1
  Mux/1 -> Out1/1

== system TestFilter/Position-Attitude Filter/Position/Attitude Filter/Position  Complementary Filter/Subsystem ==
  Euler_hat : Inport  Orientation=left
  Integer Delay2 : simulink/Discrete/Integer Delay  Orientation=left  vinit=0.0  samptime=-1  NumDelays=1
  LTP2B : dspmtrx3/Transpose  Orientation=left  SystemSampleTime=-1  Hermitian=off  overflowFlag=off
  RB2LTP : Subsystem  Orientation=left
  RB2LT : Outport  Orientation=left
  RLT2B : Outport  Orientation=left  Port=2
  wires:
  RB2LTP/1(Rot) -> RB2LT/1, LTP2B/1
  LTP2B/1 -> RLT2B/1
  Integer Delay2/1 -> RB2LTP/1(Euler)
  Euler_hat/1 -> Integer Delay2/1

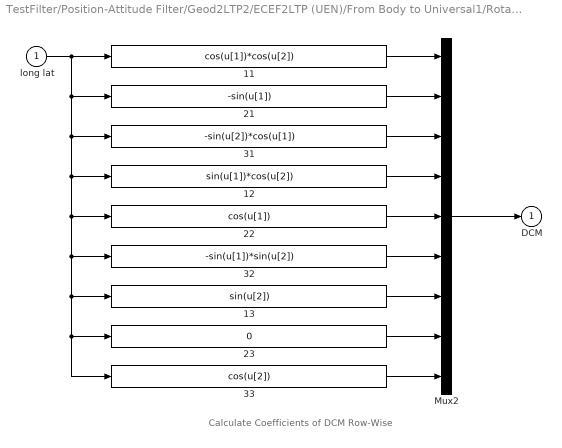
== system TestFilter/Position-Attitude Filter/Geod2LTP2/ECEF2LTP (UEN)/From Body to Universal1/Rotation Matrix from Long//Lat ==
  note: Calculate Coefficients of DCM Row-Wise
  long lat : Inport
  11 : Fcn  Expr=cos(u[1])*cos(u[2])
  12 : Fcn  Expr=sin(u[1])*cos(u[2])
  13 : Fcn  Expr=sin(u[2])
  21 : Fcn  Expr=-sin(u[1])
  22 : Fcn  Expr=cos(u[1])
  23 : Fcn  Expr=0
  31 : Fcn  Expr=-sin(u[2])*cos(u[1])
  32 : Fcn  Expr=-sin(u[1])*sin(u[2])
  33 : Fcn  Expr=cos(u[2])
  Mux2 : Mux  Inputs=9
  DCM : Outport  InitialOutput=0
  wires:
  33/1 -> Mux2/9
  23/1 -> Mux2/8
  13/1 -> Mux2/7
  32/1 -> Mux2/6
  22/1 -> Mux2/5
  12/1 -> Mux2/4
  31/1 -> Mux2/3
  21/1 -> Mux2/2
  11/1 -> Mux2/1
  Mux2/1 -> DCM/1
  long lat/1 -> 11/1, 33/1, 23/1, 13/1, 32/1, 22/1, 12/1, 31/1, 21/1

== system TestFilter/Position-Attitude Filter/Position/Attitude Filter/Attitude Complementary Filter/3vector LPF/Low Pass1 ==
  In1 : Inport
  Discrete Zero-Pole : DiscreteZeroPole  Zeros=zerosd  Poles=polesd  Gain=gaind  SampleTime=SampleTime
  Out1 : Outport
  wires:
  In1/1 -> Discrete Zero-Pole/1
  Discrete Zero-Pole/1 -> Out1/1

== system TestFilter/Position-Attitude Filter/Position/Attitude Filter/Attitude Complementary Filter/3vector LPF/Low Pass2 ==
  In1 : Inport
  Discrete Zero-Pole : DiscreteZeroPole  Zeros=zerosd  Poles=polesd  Gain=gaind  SampleTime=SampleTime
  Out1 : Outport
  wires:
  Discrete Zero-Pole/1 -> Out1/1
  In1/1 -> Discrete Zero-Pole/1

== system TestFilter/Position-Attitude Filter/Position/Attitude Filter/Attitude Complementary Filter/3vector LPF/Low Pass3 ==
  In1 : Inport
  Discrete Zero-Pole : DiscreteZeroPole  Zeros=zerosd  Poles=polesd  Gain=gaind  SampleTime=SampleTime
  Out1 : Outport
  wires:
  In1/1 -> Discrete Zero-Pole/1
  Discrete Zero-Pole/1 -> Out1/1

== system TestFilter/Position-Attitude Filter/Position/Attitude Filter/Attitude Complementary Filter/Compute Euler/Enabled Subsystem ==
  In1 : Inport
  Enable : EnablePort
  Out1 : Outport
  wires:
  In1/1 -> Out1/1

== system TestFilter/Position-Attitude Filter/Position/Attitude Filter/Attitude Complementary Filter/Compute Euler/Get COG ==
  Vn : Inport
  Ve : Inport  Port=2
  C Function Call : dsPICdrivers/OTHERS/C Function Call  Tag=dsPIC_dsPIC_CFunctionCall  fctName='myAtan2'  INPUT_SIZE=1  INPUT1=real32  INPUT2=real32  INPUT3=--  OUTPUT_SIZE=1  OUTPUT1=real32  SampleTime=-1  InputType=[ 7 7 ]  OutputType=[ 7 ]  FctDeclaration=extern real32_T myAtan2(real32_T u1, real32_T u2);  FctCall=%y1 = myAtan2(%u1, %u2);  OrderingInOutPopup=None
  Compare To Zero : simulink/Logic and Bit Operations/Compare To Zero  SystemSampleTime=-1  relop=<  LogicOutDataTypeMode=boolean  ZeroCross=off
  Data Type Conversion : DataTypeConversion  OutDataTypeMode=single
  Data Type Conversion1 : DataTypeConversion  OutDataTypeMode=single
  Data Type Conversion2 : DataTypeConversion  OutDataTypeMode=double
  Greater than or equal to zero : Subsystem  TreatAsAtomicUnit=on
  Logical Operator : Logic  Operator=NOT  AllPortsSameDT=off  OutDataTypeMode=Boolean
  Merge : Merge
  less than zero : Subsystem  TreatAsAtomicUnit=on
  COG : Outport
  wires:
  Ve/1 -> Data Type Conversion/1
  Vn/1 -> Data Type Conversion1/1
  C Function Call/1 -> Compare To Zero/1, Greater than or equal to zero/1(In1), less than zero/1(In1)
  Merge/1 -> Data Type Conversion2/1
  Compare To Zero/1 -> Logical Operator/1, less than zero/Enable
  Logical Operator/1 -> Greater than or equal to zero/Enable
  Greater than or equal to zero/1(Out1) -> Merge/1
  less than zero/1(Out1) -> Merge/2
  Data Type Conversion/1 -> C Function Call/1
  Data Type Conversion1/1 -> C Function Call/2
  Data Type Conversion2/1 -> COG/1

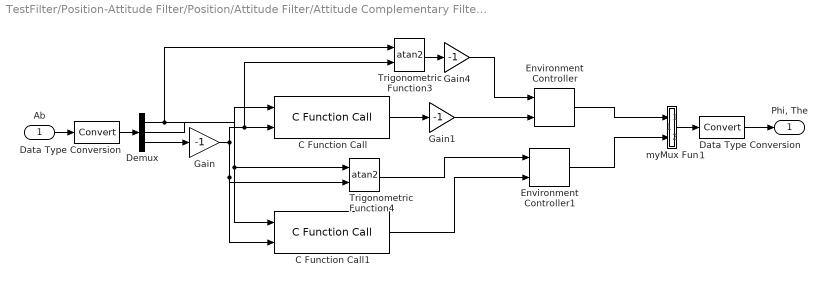
== system TestFilter/Position-Attitude Filter/Position/Attitude Filter/Attitude Complementary Filter/Compute Euler/Get Roll, Pitch ==
  Ab : Inport
  C Function Call : dsPICdrivers/OTHERS/C Function Call  Tag=dsPIC_dsPIC_CFunctionCall  fctName='myAtan2'  INPUT_SIZE=1  INPUT1=real32  INPUT2=real32  INPUT3=--  OUTPUT_SIZE=1  OUTPUT1=real32  SampleTime=-1  InputType=[ 7 7 ]  OutputType=[ 7 ]  FctDeclaration=extern real32_T myAtan2(real32_T u1, real32_T u2);  FctCall=%y1 = myAtan2(%u1, %u2);  OrderingInOutPopup=None
  C Function Call1 : dsPICdrivers/OTHERS/C Function Call  Tag=dsPIC_dsPIC_CFunctionCall  fctName='myAtan2'  INPUT_SIZE=1  INPUT1=real32  INPUT2=real32  INPUT3=--  OUTPUT_SIZE=1  OUTPUT1=real32  SampleTime=-1  InputType=[ 7 7 ]  OutputType=[ 7 ]  FctDeclaration=extern real32_T myAtan2(real32_T u1, real32_T u2);  FctCall=%y1 = myAtan2(%u1, %u2);  OrderingInOutPopup=None
  Data Type Conversion : DataTypeConversion  OutDataTypeMode=single
  Data Type Conversion1 : DataTypeConversion  OutDataTypeMode=double
  Demux : Demux  Outputs=3
  Environment Controller : simulink/Signal Routing/Environment Controller  SystemSampleTime=-1
  Environment Controller1 : simulink/Signal Routing/Environment Controller  SystemSampleTime=-1
  Gain : Gain  Gain=-1
  Gain1 : Gain  Gain=-1
  Gain4 : Gain  Gain=-1
  Trigonometric Function3 : Trigonometry  Operator=atan2  SampleTime=T
  Trigonometric Function4 : Trigonometry  Operator=atan2  SampleTime=T
  myMux Fun : Stateflow chart
  "Phi, The" : Outport
  wires:
  Ab/1 -> Data Type Conversion/1
  Demux/3 -> Gain/1
  Gain/1 -> C Function Call/2, Trigonometric Function3/2, C Function Call1/2, Trigonometric Function4/2
  Demux/2 -> C Function Call/1
  Gain1/1 -> Environment Controller/2
  Demux/1 -> Trigonometric Function3/1, C Function Call1/1, Trigonometric Function4/1
  myMux Fun/1(y) -> Data Type Conversion1/1
  C Function Call/1 -> Gain1/1
  Data Type Conversion/1 -> Demux/1
  Data Type Conversion1/1 -> "Phi, The"/1
  C Function Call1/1 -> Environment Controller1/2
  Environment Controller1/1 -> myMux Fun/2(u2)
  Environment Controller/1 -> myMux Fun/1(u1)
  Trigonometric Function3/1 -> Gain4/1
  Gain4/1 -> Environment Controller/1
  Trigonometric Function4/1 -> Environment Controller1/1

== system TestFilter/Position-Attitude Filter/Position/Attitude Filter/Attitude Complementary Filter/Compute Euler/get Centripetal ==
  pqr : Inport  Orientation=left
  Vb : Inport  Orientation=left  Port=2
  3vector LPF : Subsystem  Orientation=left  mask{flpf=100}
      mask prompts: flpf "LowPass Freq"
      mask Display: droots([],-flpf,flpf)
  3x3 Cross Product : aerolibutil/3x3 Cross Product  Orientation=left  SystemSampleTime=-1
  Integer Delay : simulink/Discrete/Integer Delay  Orientation=left  vinit=0.0  samptime=-1  NumDelays=1
  Saturation : Saturate  Orientation=left  UpperLimit=20  LowerLimit=-20
  w x Vb : Outport  Orientation=left
  wires:
  Integer Delay/1 -> 3x3 Cross Product/2
  pqr/1 -> 3vector LPF/1(In1)
  Vb/1 -> Integer Delay/1
  3x3 Cross Product/1 -> Saturation/1  "w x Vb"
  3vector LPF/1(Out1) -> 3x3 Cross Product/1
  Saturation/1 -> w x Vb/1

== system TestFilter/Position-Attitude Filter/Position/Attitude Filter/Position  Complementary Filter/3vector LPF/Low Pass1 ==
  In1 : Inport
  Discrete Zero-Pole : DiscreteZeroPole  Zeros=zerosd  Poles=polesd  Gain=gaind  SampleTime=SampleTime
  Out1 : Outport
  wires:
  In1/1 -> Discrete Zero-Pole/1
  Discrete Zero-Pole/1 -> Out1/1
